simulink model "mpc_2input_simulink"  (R2023b)
settings: Solver=VariableStepAuto  StartTime=0.0  StopTime=tsim  RelTol=1e-3
values from neighbouring files (symbols this model uses):
  A = [-a_til(2:end)' [eye(length(a_til)-2); zeros(1,length(a_til)-2)]]    [mpc_TISO.m]    (also in mpc_TISO_quadprog.m)
  B1 = [b1_til(2:end)']    [mpc_TISO.m]    (also in mpc_TISO_quadprog.m)
  B2 = [b2_til(2:end)']    [mpc_TISO.m]    (also in mpc_TISO_quadprog.m)
  D = [c(2:end)'-a_til(2:end)']    [mpc_TISO.m]    (also in mpc_TISO_quadprog.m)
  H = [1 zeros(1,Max-1)]    [mpc_TISO.m]    (also in mpc_TISO_quadprog.m)
  K = [K1*F; K2*F]    [mpc_TISO.m]
  Ke = [K1*E; K2*E]    [mpc_TISO.m]
  Kr = [K1r; K2r]    [mpc_TISO.m]
  Kur = [K3_; K3]    [mpc_TISO.m]
  r = cond_desej - cond_inicial    (= 1)    [mpc_TISO.m]    (also in mpc_TISO_quadprog.m)
  t_r = 0*Ts    (= 0)    [mpc_TISO.m]    (also in mpc_TISO_quadprog.m = 240)
  t_ur = ceil(qntd_k/2)*Ts    [mpc_TISO.m]    (also in mpc_TISO_quadprog.m)
  Ts = 24    [mpc_TISO.m]    (also in mpc_TISO_quadprog.m)
  tsim = qntd_k*Ts    (= 5400)    [mpc_TISO.m]    (also in mpc_TISO_quadprog.m)
  ur = 1    [mpc_TISO.m]    (also in mpc_TISO_quadprog.m)
undefined symbols (not defined in the file or in its folder): Delta, temp_atual
libraries: cstblocks x3
settings Model: Creator=junio  LastModifiedBy=sergio

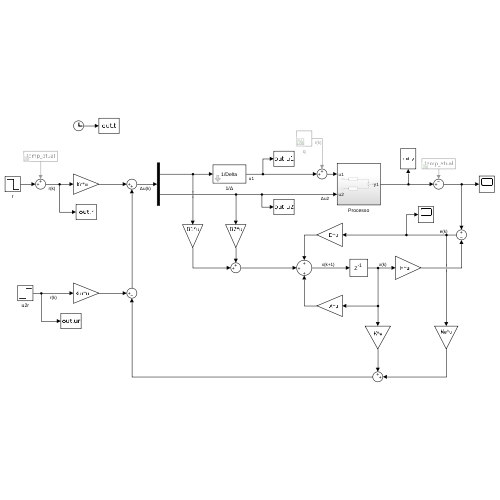
[thumbnail: Simulink's stored preview of the top-level diagram]
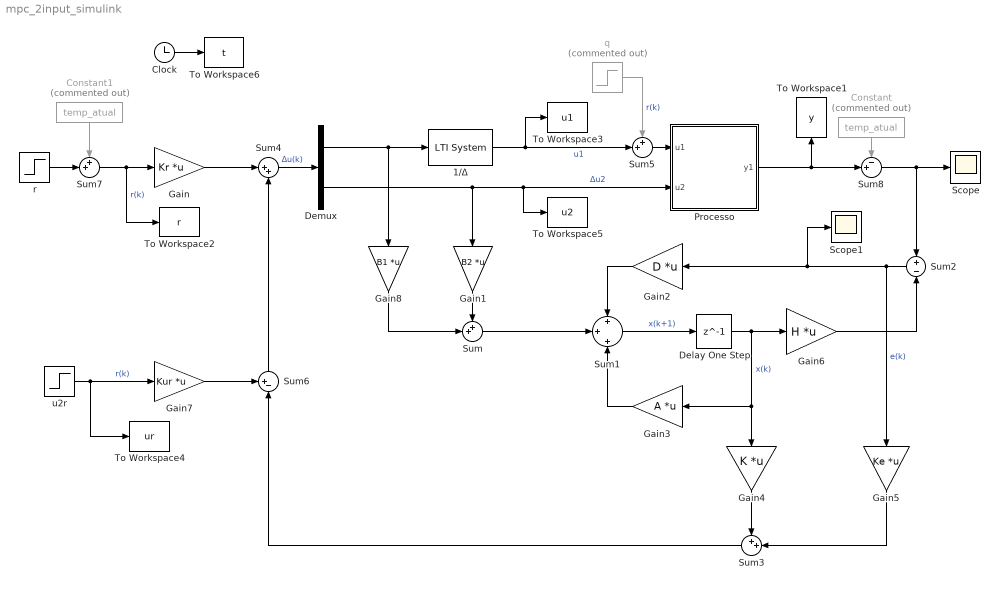
== system mpc_2input_simulink ==
  1/Δ : cstblocks/LTI System  sys=1/Delta  IC=[]  PadeOrder=0
  Clock : Clock
  Constant : Constant  Commented=on  Value=temp_atual  SampleTime=Ts
  Constant1 : Constant  Commented=on  Value=temp_atual  SampleTime=Ts
  Delay One Step : Delay  DelayLength=1
  Demux : Demux  Outputs=2
  Gain : Gain  Gain=Kr  Multiplication=Matrix(K*u)
  Gain1 : Gain  Gain=B2  Multiplication=Matrix(K*u)
  Gain2 : Gain  Gain=D  Multiplication=Matrix(K*u)
  Gain3 : Gain  Gain=A  Multiplication=Matrix(K*u)
  Gain4 : Gain  Gain=K  Multiplication=Matrix(K*u)
  Gain5 : Gain  Gain=Ke  Multiplication=Matrix(K*u)
  Gain6 : Gain  Gain=H  Multiplication=Matrix(K*u)
  Gain7 : Gain  Gain=Kur  Multiplication=Matrix(K*u)
  Gain8 : Gain  Gain=B1  Multiplication=Matrix(K*u)
  Processo : Subsystem
  Scope : Scope
  Scope1 : Scope
  Sum{,3,5,7} (4 alike) : Sum  Inputs=++|
  Sum1 : Sum  Inputs=+|+|+
  Sum2 : Sum  Inputs=+|-
  Sum4 : Sum  Inputs=|++
  Sum6 : Sum  Inputs=+-|
  Sum8 : Sum  Inputs=-+|
  To Workspace1 : ToWorkspace  VariableName=y  SampleTime=Ts
      settings: Save2DSignal=2-D array (concatenate along first dimension)
  To Workspace2 : ToWorkspace  VariableName=r  SampleTime=Ts
      settings: Save2DSignal=2-D array (concatenate along first dimension)
  To Workspace3 : ToWorkspace  VariableName=u1  SampleTime=Ts
      settings: Save2DSignal=2-D array (concatenate along first dimension)
  To Workspace4 : ToWorkspace  VariableName=ur  SampleTime=Ts
      settings: Save2DSignal=2-D array (concatenate along first dimension)
  To Workspace5 : ToWorkspace  VariableName=u2  SampleTime=Ts
      settings: Save2DSignal=2-D array (concatenate along first dimension)
  To Workspace6 : ToWorkspace  VariableName=t  SampleTime=Ts
      settings: Save2DSignal=2-D array (concatenate along first dimension)
  q : Step  Commented=on  Time=tsim/2  After=-1  SampleTime=Ts
  r : Step  Time=t_r  After=r  SampleTime=Ts
  u2r : Step  Time=t_ur  After=ur  SampleTime=Ts
  wires:
  Gain2/1 -> Sum1/1
  Gain3/1 -> Sum1/3
  Sum1/1 -> Delay One Step/1  "x(k+1)"
  Delay One Step/1 -> Gain6/1, Gain4/1, Gain3/1  "x(k)"
  Sum2/1 -> Scope1/1, Gain2/1, Gain5/1  "e(k)"
  Gain6/1 -> Sum2/2
  Gain4/1 -> Sum3/1
  Gain5/1 -> Sum3/2
  Gain/1 -> Sum4/1
  u2r/1 -> To Workspace4/1, Gain7/1  "r(k)"
  Gain7/1 -> Sum6/1
  Sum3/1 -> Sum6/2
  Sum4/1 -> Demux/1  "Δu(k)"
  Demux/1 -> Gain8/1, 1/Δ/1
  1/Δ/1 -> Sum5/2, To Workspace3/1  "u1"
  Sum/1 -> Sum1/2
  Gain1/1 -> Sum/1
  Gain8/1 -> Sum/2
  Sum8/1 -> Sum2/1, Scope/1
  Demux/2 -> Processo/2(u2), To Workspace5/1, Gain1/1  "Δu2"
  Clock/1 -> To Workspace6/1
  Sum7/1 -> Gain/1, To Workspace2/1  "r(k)"
  Sum6/1 -> Sum4/2
  Sum5/1 -> Processo/1(u1)
  q/1 -> Sum5/1  "r(k)"
  Processo/1(y1) -> To Workspace1/1, Sum8/2
  Constant/1 -> Sum8/1
  r/1 -> Sum7/2
  Constant1/1 -> Sum7/1

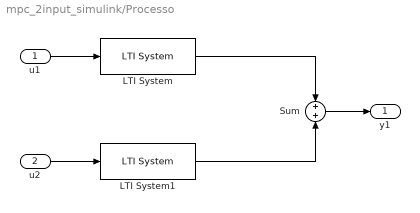
== system mpc_2input_simulink/Processo ==
  u1 : Inport
  u2 : Inport  Port=2
  LTI System : cstblocks/LTI System  sys=Gz1  IC=[]  PadeOrder=0
  LTI System1 : cstblocks/LTI System  sys=Gz2  IC=[]  PadeOrder=0
  Sum : Sum  Inputs=+|+
  y1 : Outport
  wires:
  u2/1 -> LTI System1/1
  u1/1 -> LTI System/1
  Sum/1 -> y1/1
  LTI System/1 -> Sum/1
  LTI System1/1 -> Sum/2
